simulink model "SCARA_215_ozk"  (R2015a)
settings: Solver=ode1  StartTime=0.0  StopTime=Inf  FixedStep=0.001  RelTol=1e-3
PostLoadFcn:
  | , if any(exist('dsrtsu_mdlpostloadfcn', 'file') == [2, 3, 6]), try dsrtsu_mdlpostloadfcn('Execute', bdroot); catch fprintf('Error in PostLoadFcn (dsrtsu_mdlpostloadfcn) for model "%s":\n %s\n', bdroot, lasterr); end, end,
libraries: rtilib1104 x9, simulink x7, simulink_extras x2
settings Model: DSRTSU_INTERNAL_RTI_VER=460  DSRTSU_INTERNAL_RTI_TYPE=rti1104  DSRTSU_INTERNAL_RTIFPGA=50  Creator=k18p800a  LastModifiedBy=k18p800a
settings OptimizationCC: BlockReduction=off  OptimizeBlockIOStorage=off  BufferReuse=off  GlobalBufferReuse=off  ExpressionFolding=off  LocalBlockOutputs=off
settings HardwareCC: ProdIntDivRoundTo=Zero  ProdEndianess=BigEndian  ProdHWDeviceType=Generic->Custom  TargetIntDivRoundTo=Zero  TargetEndianess=BigEndian  TargetHWDeviceType=Generic->Custom
settings RTWCC: SystemTargetFile=rti1104.tlc  MakeCommand=make_rti  TemplateMakefile=rti1104.tmf  Description=dSPACE DS1104 Hardware Platform
settings STFCustomTargetCC: GenerateSampleERTMain=off  ParMdlRefBuildCompliant=on  GeneratePreprocessorConditionals=Disable all  ERTCustomFileBanners=off  SupportNonInlinedSFcns=on  SupportVariableSizeSignals=off  MATLABClassNameForMDSCustomization=Simulink.SoftwareTarget.GRTCustomization  GRTInterface=on  SystemTargetFile=rti1104.tlc
settings GRTTargetCC: CompOptLevelCompliant=off  ConcurrentExecutionCompliant=off  CombineOutputUpdateFcns=off  MatFileLogging=off  CPPClassGenCompliant=off  GRTInterface=on  ExtModeMexFile=noextcomm

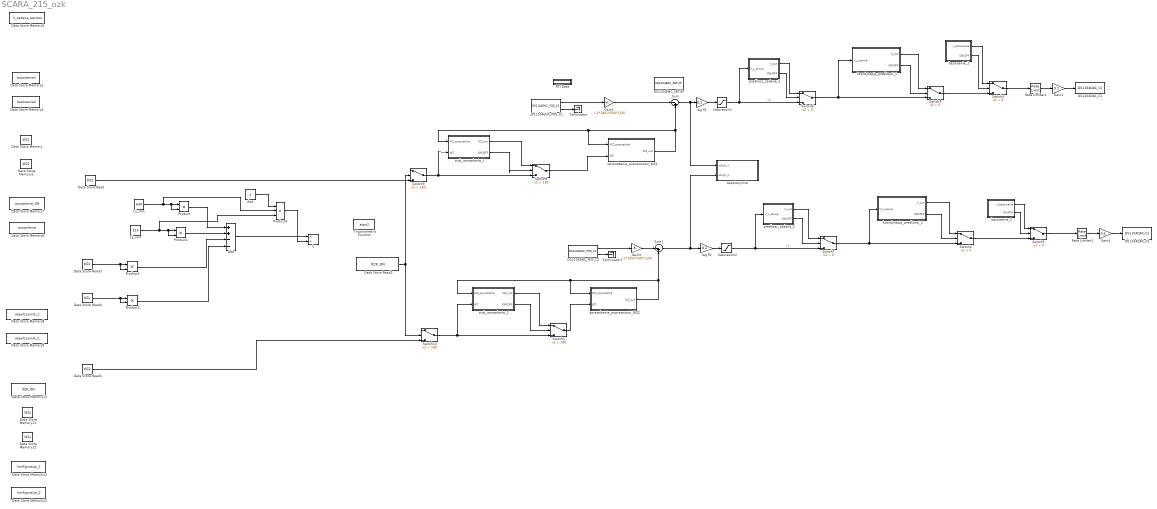
== system SCARA_215_ozk ==
  Add : Sum  Inputs=++--
  DS1104DAC_C1 : rtilib1104/DS1104 MASTER PPC/DS1104DAC_C1  ChannelNo=1  InitValue=0  TermMode=0  TermValue=0  Reserved1=[]  Reserved2=[]  Reserved3=[]  Reserved4=[]  DialogFcn=gui1104dac  UnitName={ 'DS1104DAC_C'}  UnitValues={ 1 }  DSProperties=struct('RTI',struct('Version',uint32(1),'BlockType',struct('isSLSource',uint8(0),'isSLSink',uint8(1),'isHWSource',uint8(0),'isHWSink',uint8(1),'isSetup',uint8(0),'isInline',uint8(1),'isNonInline',uint8(0),'isInterrupt',uint8(0),'isChannelwise',uint8(1)),'IOBoardType','DS1104MASTER','UnitType','DAC','Identifier','DAC','DialogType','ML','BlockSet','NONE','SlaveProcessor','NONE'))
  DS1104DAC_C2 : rtilib1104/DS1104 MASTER PPC/DS1104DAC_C1  ChannelNo=2  InitValue=0  TermMode=0  TermValue=0  Reserved1=[]  Reserved2=[]  Reserved3=[]  Reserved4=[]  DialogFcn=gui1104dac  UnitName={ 'DS1104DAC_C'}  UnitValues={2}  DSProperties=struct('RTI',struct('Version',uint32(1),'BlockType',struct('isSLSource',uint8(0),'isSLSink',uint8(1),'isHWSource',uint8(0),'isHWSink',uint8(1),'isSetup',uint8(0),'isInline',uint8(1),'isNonInline',uint8(0),'isInterrupt',uint8(0),'isChannelwise',uint8(1)),'IOBoardType','DS1104MASTER','UnitType','DAC','Identifier','DAC','DialogType','ML','BlockSet','NONE','SlaveProcessor','NONE'))
  DS1104ENC_POS_C2 : rtilib1104/DS1104 MASTER PPC/DS1104ENC_POS_C1  ChannelNo=2  PosValue=0  Reserved1=[]  Reserved2=[]  Reserved3=[]  Reserved4=[]  DialogFcn=gui1104enc_pos  UnitName={'DS1104ENC_POS_C'}  UnitValues={ 2 }  DSProperties=struct('RTI',struct('Version',uint32(1),'BlockType',struct('isSLSource',uint8(1),'isSLSink',uint8(0),'isHWSource',uint8(1),'isHWSink',uint8(0),'isSetup',uint8(0),'isInline',uint8(1),'isNonInline',uint8(0),'isInterrupt',uint8(0),'isChannelwise',uint8(1)),'IOBoardType','DS1104MASTER','UnitType','ENC','Identifier','ENCPOSCH','DialogType','ML','BlockSet','NONE','SlaveProcessor','NONE'))
  DS1104ENC_SETUP : rtilib1104/DS1104 MASTER PPC/DS1104ENC_SETUP  Reserved1=[]  Reserved2=[]  Reserved3=[]  Reserved4=[]  DialogFcn=gui1104enc_setup  UnitName={'DS1104ENC_SETUP'}  UnitValues={ [] }  DSProperties=struct('RTI',struct('Version',uint32(1),'BlockType',struct('isSLSource',uint8(0),'isSLSink',uint8(0),'isHWSource',uint8(0),'isHWSink',uint8(0),'isSetup',uint8(0),'isInline',uint8(1),'isNonInline',uint8(0),'isInterrupt',uint8(0),'isChannelwise',uint8(0)),'IOBoardType','DS1104MASTER','UnitType','ENC','Identifier','ENCSETUP','DialogType','ML','BlockSet','NONE','SlaveProcessor','NONE'))
      settings: SignalType=[0 0]
  Data Store Memory : DataStoreMemory  DataStoreName=WZ1  ReadBeforeWriteMsg=warning  WriteAfterWriteMsg=warning  WriteAfterReadMsg=warning
  Data Store Memory1 : DataStoreMemory  DataStoreName=WZ2  ReadBeforeWriteMsg=warning  WriteAfterWriteMsg=warning  WriteAfterReadMsg=warning
  Data Store Memory11 : DataStoreMemory  DataStoreName=WZx  ReadBeforeWriteMsg=warning  WriteAfterWriteMsg=warning  WriteAfterReadMsg=warning
  Data Store Memory12 : DataStoreMemory  DataStoreName=WZy  ReadBeforeWriteMsg=warning  WriteAfterWriteMsg=warning  WriteAfterReadMsg=warning
  Data Store Memory13 : DataStoreMemory  DataStoreName=OZK_ON  ReadBeforeWriteMsg=warning  WriteAfterWriteMsg=warning  WriteAfterReadMsg=warning  InitialValue=false  OutDataTypeStr=boolean
  Data Store Memory14 : DataStoreMemory  DataStoreName=konfiguracja_1  ReadBeforeWriteMsg=warning  WriteAfterWriteMsg=warning  WriteAfterReadMsg=warning  InitialValue=false  OutDataTypeStr=boolean
  Data Store Memory15 : DataStoreMemory  DataStoreName=konfiguracja_2  ReadBeforeWriteMsg=warning  WriteAfterWriteMsg=warning  WriteAfterReadMsg=warning  InitialValue=false  OutDataTypeStr=boolean
  Data Store Memory2 : DataStoreMemory  DataStoreName=bazowanie1  ReadBeforeWriteMsg=warning  WriteAfterWriteMsg=warning  WriteAfterReadMsg=warning  InitialValue=false  OutDataTypeStr=boolean
  Data Store Memory3 : DataStoreMemory  DataStoreName=bazowanie2  ReadBeforeWriteMsg=warning  WriteAfterWriteMsg=warning  WriteAfterReadMsg=warning  InitialValue=false  OutDataTypeStr=boolean
  Data Store Memory5 : DataStoreMemory  DataStoreName=V_zadana_wartosc  ReadBeforeWriteMsg=warning  WriteAfterWriteMsg=warning  WriteAfterReadMsg=warning  InitialValue=100  OutDataTypeStr=double
  Data Store Memory6 : DataStoreMemory  DataStoreName=wyzwolenie  ReadBeforeWriteMsg=warning  WriteAfterWriteMsg=warning  WriteAfterReadMsg=warning  InitialValue=false  OutDataTypeStr=boolean
  Data Store Memory7 : DataStoreMemory  DataStoreName=wyzwalanie_ON  ReadBeforeWriteMsg=warning  WriteAfterWriteMsg=warning  WriteAfterReadMsg=warning  InitialValue=false  OutDataTypeStr=boolean
  Data Store Memory8 : DataStoreMemory  DataStoreName=wspolczynnik_1  ReadBeforeWriteMsg=warning  WriteAfterWriteMsg=warning  WriteAfterReadMsg=warning
  Data Store Memory9 : DataStoreMemory  DataStoreName=wspolczynnik_2  ReadBeforeWriteMsg=warning  WriteAfterWriteMsg=warning  WriteAfterReadMsg=warning
  Data Store Read : DataStoreRead  DialogController=Simulink.DDGSource  DataStoreName=WZ1
  Data Store Read1 : DataStoreRead  DataStoreName=WZ2
  Data Store Read2 : DataStoreRead  DataStoreName=OZK_ON
  Data Store Read3 : DataStoreRead  DataStoreName=WZx
  Data Store Read4 : DataStoreRead  DataStoreName=WZy
  Gain1 : Gain  Gain=(-2*180)/(500*128)
  Gain2 : Gain  Gain=0.1
  Gain3 : Gain  Gain=(-2*180)/(500*128)
  Gain4 : Gain  Gain=0.1
  L : Product  Inputs=*/
  L1_mm : Constant  Value=630
  "L2_mm " : Constant  Value=510
  Product{,1..3} (4 alike) : Product
  Product4 : Product  Inputs=3
  RTI Data : Subsystem  Tag=struct('RTIDataServer',struct('RTIDataServerVs','2','RTIModelDescription','struct(''main'',''SCARA_215_ozk'',''sub'',''SCARA_215_ozk'',''isMp'',0)'))  LoadFcn="if exist('rtidc'), try,  rtidc('DataHostBlockClbLoad', gcbh); catch, disp(['Warning: ''LoadFcn'' for RTI Data block failed: ' lasterr]); end, end,"  mask(RTI_DATA_HOST){}
      mask help:
      | RTI Data Block.
      | This block is used by RTI to store internal model-dependent data.
      | Please keep this block on the root level of the model. Deleting this block will result in data loss.
      |
      | NEVER DELETE OR COPY THIS BLOCK!
      settings: CopyFcn="if exist('rtidc'), try,  rtidc('DataHostBlockClbCopy', gcbh); catch, disp(['Warning: ''CopyFcn'' for RTI Data block failed: ' lasterr]); end, end,"  DeleteFcn="if exist('rtidc'), try,  rtidc('DataHostBlockClbDelete', gcbh); catch, disp(['Warning: ''DeleteFcn'' for RTI Data block failed: ' lasterr]); end, end,"  ModelCloseFcn="if exist('rtidc'), try,  rtidc('DataHostBlockClbModelClose', gcbh); catch, disp(['Warning: ''ModelCloseFcn'' for RTI Data block failed: ' lasterr]); end, end,"  PreSaveFcn="if exist('rtidc'), try,  rtidc('DataHostBlockClbPreSave', gcbh); catch, disp(['Warning: ''PreSaveFcn'' for RTI Data block failed: ' lasterr]); end, end,"  PostSaveFcn="if exist('rtidc'), try,  rtidc('DataHostBlockClbPostSave', gcbh); catch, disp(['Warning: ''PostSaveFcn'' for RTI Data block failed: ' lasterr]); end, end,"  NameChangeFcn="if exist('rtidc'), try,  rtidc('DataHostBlockClbNameChange', gcbh); catch, disp(['Warning: ''NameChangeFcn'' for RTI Data block failed: ' lasterr]); end, end,"
      mask Help:
      | RTI Data Block.
      | This block is used by RTI to store internal model-dependent data.
      | Please keep this block on the root level of the model. Deleting this block will result in data loss.
      | 
      | NEVER DELETE OR COPY THIS BLOCK!
      mask Display:
      | text(0.5, 0.5, 'RTI Data', 'HorizontalAlignment', 'center');
      | plot([1 0]);
  Rate Limiter1 : RateLimiter  RisingSlewLimit=50  FallingSlewLimit=-50  SampleTimeMode=inherited
  Rate Limiter2 : RateLimiter  RisingSlewLimit=50  FallingSlewLimit=-50  SampleTimeMode=inherited
  Saturation1 : Saturate  UpperLimit=3  LowerLimit=-3
  Saturation2 : Saturate  UpperLimit=3  LowerLimit=-3
  Sum : Sum  Inputs=|-+
  Sum1 : Sum  Inputs=|-+
  Switch{1,8..10} (4 alike) : Switch  Criteria=u2 > Threshold  Threshold=180
  Switch{2..7} (6 alike) : Switch  Criteria=u2 > Threshold
  Terminator : Terminator
  Terminator1 : Terminator
  Trigonometric Function : Trigonometry  Operator=atan2
  _DS1104ENC_POS_C1 : rtilib1104/DS1104 MASTER PPC/DS1104ENC_POS_C1  ChannelNo=1  PosValue=0  Reserved1=[]  Reserved2=[]  Reserved3=[]  Reserved4=[]  DialogFcn=gui1104enc_pos  UnitName={'DS1104ENC_POS_C'}  UnitValues={ 1 }  DSProperties=struct('RTI',struct('Version',uint32(1),'BlockType',struct('isSLSource',uint8(1),'isSLSink',uint8(0),'isHWSource',uint8(1),'isHWSink',uint8(0),'isSetup',uint8(0),'isInline',uint8(1),'isNonInline',uint8(0),'isInterrupt',uint8(0),'isChannelwise',uint8(1)),'IOBoardType','DS1104MASTER','UnitType','ENC','Identifier','ENCPOSCH','DialogType','ML','BlockSet','NONE','SlaveProcessor','NONE'))
  bazowanie_1 : Subsystem
  "bazowanie_2 " : Subsystem
  dwa : Constant  Value=2
  koordynacja_predkosci_1 : Subsystem
  koordynacja_predkosci_2 : Subsystem
  predkosc_zadana_1 : Subsystem
  predkosc_zadana_2 : Subsystem
  reg P1 : Gain  Gain=0.2
  reg P2 : Gain  Gain=0.2
  sprawdzenie_poprawnosci_WZ1 : Subsystem
  sprawdzenie_poprawnosci_WZ2 : Subsystem
  tryb_wyzwalania_1 : Subsystem
  tryb_wyzwalania_2 : Subsystem
  wspolczynniki : Subsystem
  wires:
  Rate Limiter1/1 -> Gain2/1
  Rate Limiter2/1 -> Gain4/1
  reg P1/1 -> Saturation1/1
  reg P2/1 -> Saturation2/1
  Sum/1 -> wspolczynniki/1(uchyb_1), reg P1/1
  Sum1/1 -> wspolczynniki/2(uchyb_2), reg P2/1
  _DS1104ENC_POS_C1/1 -> Gain1/1
  Gain1/1 -> Sum/1
  DS1104ENC_POS_C2/1 -> Gain3/1
  Gain3/1 -> Sum1/1
  Gain2/1 -> DS1104DAC_C1/1
  Gain4/1 -> DS1104DAC_C2/1
  _DS1104ENC_POS_C1/2 -> Terminator/1
  DS1104ENC_POS_C2/2 -> Terminator1/1
  Switch4/1 -> Rate Limiter1/1
  Switch5/1 -> Rate Limiter2/1
  bazowanie_1/1(v_bazowania) -> Switch4/1
  bazowanie_1/2(ON/OFF) -> Switch4/2
  "bazowanie_2 "/1(v_bazowania) -> Switch5/1
  "bazowanie_2 "/2(On/OFF) -> Switch5/2
  Saturation1/1 -> predkosc_zadana_1/1(V_z_serwa), Switch6/3  "v1"
  predkosc_zadana_1/1(V_out) -> Switch6/1
  predkosc_zadana_1/2(ON/OFF) -> Switch6/2
  Saturation2/1 -> Switch7/3, predkosc_zadana_2/1(V_z_serwa)  "v1"
  predkosc_zadana_2/1(V_out) -> Switch7/1
  predkosc_zadana_2/2(ON/OFF) -> Switch7/2
  tryb_wyzwalania_1/1(WZ_out) -> Switch8/1
  tryb_wyzwalania_1/2(ON/OFF) -> Switch8/2
  sprawdzenie_poprawnosci_WZ1/1(WZ_out) -> Sum/2, tryb_wyzwalania_1/1(WZ_poprzednia), sprawdzenie_poprawnosci_WZ1/1(WZ_poprzednia)
  Switch8/1 -> sprawdzenie_poprawnosci_WZ1/2(WZ)
  tryb_wyzwalania_2/1(WZ_out) -> Switch1/1
  tryb_wyzwalania_2/2(ON/OFF) -> Switch1/2
  sprawdzenie_poprawnosci_WZ2/1(WZ_out) -> Sum1/2, tryb_wyzwalania_2/1(WZ_poprzednia), sprawdzenie_poprawnosci_WZ2/1(WZ_poprzednia)
  Switch1/1 -> sprawdzenie_poprawnosci_WZ2/2(WZ)
  Switch2/1 -> Switch5/3
  Switch7/1 -> koordynacja_predkosci_2/1(V_z_serwa), Switch2/3
  koordynacja_predkosci_2/1(V_out) -> Switch2/1
  koordynacja_predkosci_2/2(ON/OFF) -> Switch2/2
  Switch3/1 -> Switch4/3
  Switch6/1 -> koordynacja_predkosci_1/1(V_z_serwa), Switch3/3
  koordynacja_predkosci_1/1(V_out) -> Switch3/1
  koordynacja_predkosci_1/2(ON/OFF) -> Switch3/2
  Switch9/1 -> tryb_wyzwalania_1/2(WZ), Switch8/3
  Data Store Read/1 -> Switch9/3
  Switch10/1 -> tryb_wyzwalania_2/2(WZ), Switch1/3
  Data Store Read1/1 -> Switch10/3
  Data Store Read2/1 -> Switch9/2, Switch10/2
  L1_mm/1 -> Product4/2, Product/2, Product/1
  "L2_mm "/1 -> Product4/3, Product1/2, Product1/1
  Data Store Read3/1 -> Product2/2, Product2/1
  Data Store Read4/1 -> Product3/2, Product3/1
  Product/1 -> Add/1
  Product1/1 -> Add/2
  Product2/1 -> Add/3
  Product3/1 -> Add/4
  Add/1 -> L/1
  dwa/1 -> Product4/1
  Product4/1 -> L/2

== system SCARA_215_ozk/RTI Data ==
  RTI Data Store : Subsystem  Tag="struct('private',struct('version',struct('dsVer',uint32(2),'dsVerCreation',uint32(2),'RTI',struct('ver','7.4','type','RTI1104')),'access',struct('type','Model','isPerm',1,'created',['26-Mar-2018 08:24:55'],'modified',['16-Apr-2018 08:48:33'],'location','')),'public',struct('main',struct('data',[]),'sub',struct('name',{{'SCARA_215_ozk'}},'data',{{struct('TH',struct('thTaskInfo',struct('taskType',{'TIMER','HWINT','TMRINT','SWINT','GLINT'},'tasksNumOf',{1,0,0,0,0},'srcIds',{{'TIMERA'},{},{},{},{}},'taskNames',{{['Timer Task 1']},{},{},{},{}})),'th_tc',struct('dataType','TASK','taskGroupId','','taskGroupList',{{}},'taskSchedulingPolicy','FCFS','taskType','TIMER','blkh',-1,'srcId','TIMERA','srcSgnName',['Timer A interrupt'],'srcCpuName','','taskName',['Timer Task 1  [0.001] s'],'taskNameDisplayExt','','smplTime',0.001,'smplTimeOffs',0,'hasFixedPriority',0,'priority',1,'hasFixedOvc',0,'ovcType',1,'ovcMax',1),'tc_th',struct('dataType','TASK','taskGroupId','','taskGroupList',{{}},'taskSchedulingPolicy','FCFS','taskType','TIMER','blkh',-1,'srcId','TIMERA','srcSgnName',['Timer A interrupt'],'srcCpuName','','taskName',['Timer Task 1  [0.001] s'],'taskNameDisplayExt','','smplTime',0.001,'smplTimeOffs',0,'hasFixedPriority',0,'priority',1,'hasFixedOvc',0,'ovcType',1,'ovcMax',1))}})))"  mask(RTI_DATA_STORE){}
      mask help:
      | RTI Data Store Block. This block is used by RTI to store internal model dependent data. Deleting this block will result in data loss.
      |
      | NEVER DELETE, COPY, OR MODIFY THIS BLOCK!
      mask Help:
      | RTI Data Store Block. This block is used by RTI to store internal model dependent data. Deleting this block will result in data loss.
      | 
      | NEVER DELETE, COPY, OR MODIFY THIS BLOCK!
      mask Display: text(0.5, 0.5, ' ', 'HorizontalAlignment', 'center');

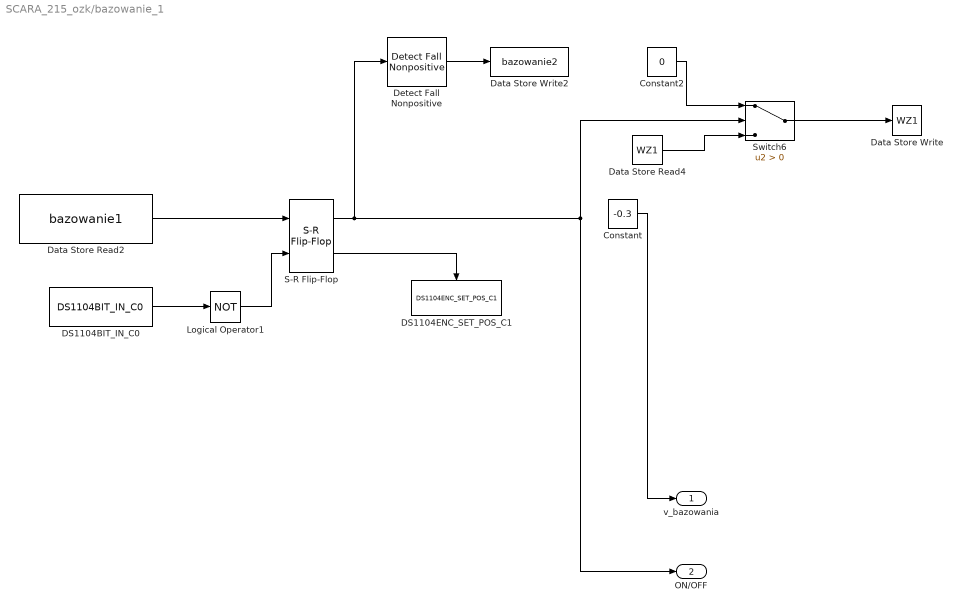
== system SCARA_215_ozk/bazowanie_1 ==
  Constant : Constant  Value=-0.3
  Constant2 : Constant  Value=0
  DS1104BIT_IN_C0 : rtilib1104/DS1104 MASTER PPC/DS1104BIT_IN_C0  ChannelNo=0  Reserved1=[]  Reserved2=[]  Reserved3=[]  Reserved4=[]  DialogFcn=gui1104bit_in  UnitName={'DS1104BIT_IN_C'}  UnitValues={ 0 }  DSProperties=struct('RTI',struct('Version',uint32(1),'BlockType',struct('isSLSource',uint8(1),'isSLSink',uint8(0),'isHWSource',uint8(1),'isHWSink',uint8(0),'isSetup',uint8(0),'isInline',uint8(1),'isNonInline',uint8(0),'isInterrupt',uint8(0),'isChannelwise',uint8(1)),'IOBoardType','DS1104MASTER','UnitType','BIT','Identifier','BITINCH','DialogType','ML','BlockSet','NONE','SlaveProcessor','NONE'))
  DS1104ENC_SET_POS_C1 : rtilib1104/DS1104 MASTER PPC/DS1104ENC_SET_POS_C1  ChannelNo=1  PosValue=0  Reserved1=[]  Reserved2=[]  Reserved3=[]  Reserved4=[]  DialogFcn=gui1104enc_set_pos  UnitName={'DS1104ENC_SET_POS_C'}  UnitValues={ 1 }  DSProperties=struct('RTI',struct('Version',uint32(1),'BlockType',struct('isSLSource',uint8(0),'isSLSink',uint8(1),'isHWSource',uint8(0),'isHWSink',uint8(1),'isSetup',uint8(0),'isInline',uint8(1),'isNonInline',uint8(0),'isInterrupt',uint8(0),'isChannelwise',uint8(1)),'IOBoardType','DS1104MASTER','UnitType','ENC','Identifier','ENCRESET','DialogType','ML','BlockSet','NONE','SlaveProcessor','NONE'))
  Data Store Read2 : DataStoreRead  DataStoreName=bazowanie1
  Data Store Read4 : DataStoreRead  DialogController=Simulink.DDGSource  DataStoreName=WZ1
  Data Store Write : DataStoreWrite  DataStoreName=WZ1
  Data Store Write2 : DataStoreWrite  DataStoreName=bazowanie2
  Detect Fall Nonpositive : simulink/Logic and Bit Operations/Detect Fall Nonpositive  vinit=1  InputProcessing=Inherited  OutDataTypeStr=boolean
  Logical Operator1 : Logic  Operator=NOT  AllPortsSameDT=off  OutDataTypeStr=boolean
  S-R Flip-Flop : simulink_extras/Flip Flops/S-R Flip-Flop  initial_condition=0
  Switch6 : Switch  Criteria=u2 > Threshold
  v_bazowania : Outport
  ON/OFF : Outport  Port=2
  wires:
  Constant/1 -> v_bazowania/1
  S-R Flip-Flop/2 -> DS1104ENC_SET_POS_C1/Trigger
  Data Store Read2/1 -> S-R Flip-Flop/1
  S-R Flip-Flop/1 -> ON/OFF/1, Switch6/2, Detect Fall Nonpositive/1
  Logical Operator1/1 -> S-R Flip-Flop/2
  DS1104BIT_IN_C0/1 -> Logical Operator1/1
  Data Store Read4/1 -> Switch6/3
  Constant2/1 -> Switch6/1
  Switch6/1 -> Data Store Write/1
  Detect Fall Nonpositive/1 -> Data Store Write2/1

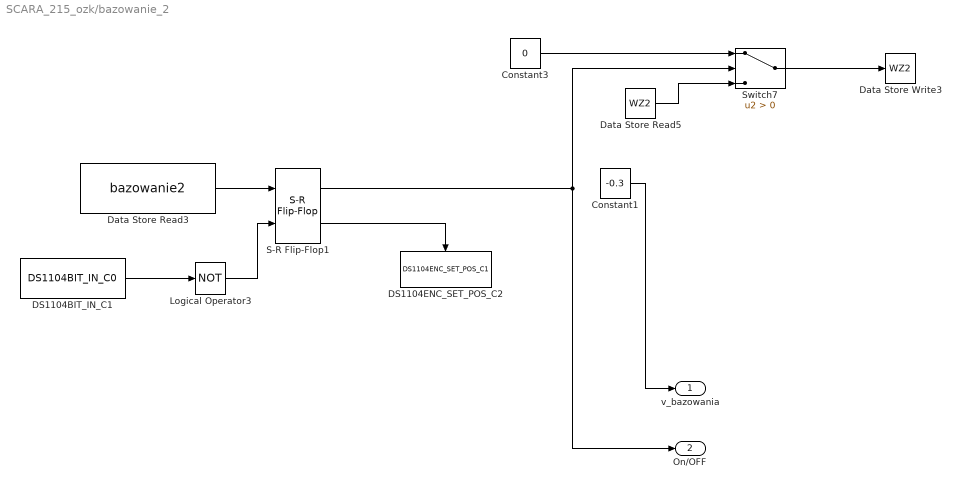
== system SCARA_215_ozk/bazowanie_2  ==
  Constant1 : Constant  Value=-0.3
  Constant3 : Constant  Value=0
  DS1104BIT_IN_C1 : rtilib1104/DS1104 MASTER PPC/DS1104BIT_IN_C0  ChannelNo=1  Reserved1=[]  Reserved2=[]  Reserved3=[]  Reserved4=[]  DialogFcn=gui1104bit_in  UnitName={'DS1104BIT_IN_C'}  UnitValues={ 1 }  DSProperties=struct('RTI',struct('Version',uint32(1),'BlockType',struct('isSLSource',uint8(1),'isSLSink',uint8(0),'isHWSource',uint8(1),'isHWSink',uint8(0),'isSetup',uint8(0),'isInline',uint8(1),'isNonInline',uint8(0),'isInterrupt',uint8(0),'isChannelwise',uint8(1)),'IOBoardType','DS1104MASTER','UnitType','BIT','Identifier','BITINCH','DialogType','ML','BlockSet','NONE','SlaveProcessor','NONE'))
  DS1104ENC_SET_POS_C2 : rtilib1104/DS1104 MASTER PPC/DS1104ENC_SET_POS_C1  ChannelNo=2  PosValue=0  Reserved1=[]  Reserved2=[]  Reserved3=[]  Reserved4=[]  DialogFcn=gui1104enc_set_pos  UnitName={'DS1104ENC_SET_POS_C'}  UnitValues={2}  DSProperties=struct('RTI',struct('Version',uint32(1),'BlockType',struct('isSLSource',uint8(0),'isSLSink',uint8(1),'isHWSource',uint8(0),'isHWSink',uint8(1),'isSetup',uint8(0),'isInline',uint8(1),'isNonInline',uint8(0),'isInterrupt',uint8(0),'isChannelwise',uint8(1)),'IOBoardType','DS1104MASTER','UnitType','ENC','Identifier','ENCRESET','DialogType','ML','BlockSet','NONE','SlaveProcessor','NONE'))
  Data Store Read3 : DataStoreRead  DataStoreName=bazowanie2
  Data Store Read5 : DataStoreRead  DialogController=Simulink.DDGSource  DataStoreName=WZ2
  Data Store Write3 : DataStoreWrite  DataStoreName=WZ2
  Logical Operator3 : Logic  Operator=NOT  AllPortsSameDT=off  OutDataTypeStr=boolean
  S-R Flip-Flop1 : simulink_extras/Flip Flops/S-R Flip-Flop  initial_condition=0
  Switch7 : Switch  Criteria=u2 > Threshold
  v_bazowania : Outport
  On/OFF : Outport  Port=2
  wires:
  Constant1/1 -> v_bazowania/1
  S-R Flip-Flop1/2 -> DS1104ENC_SET_POS_C2/Trigger
  Data Store Read3/1 -> S-R Flip-Flop1/1
  Logical Operator3/1 -> S-R Flip-Flop1/2
  DS1104BIT_IN_C1/1 -> Logical Operator3/1
  Data Store Read5/1 -> Switch7/3
  Constant3/1 -> Switch7/1
  Switch7/1 -> Data Store Write3/1
  S-R Flip-Flop1/1 -> On/OFF/1, Switch7/2

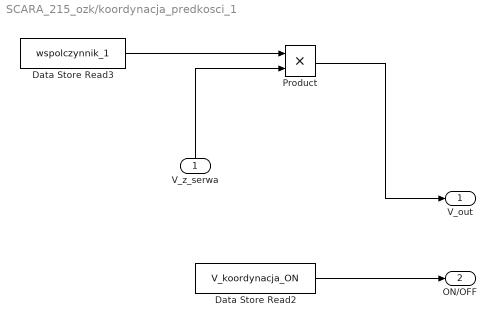
== system SCARA_215_ozk/koordynacja_predkosci_1 ==
  V_z_serwa : Inport
  Data Store Read2 : DataStoreRead  DataStoreName=V_koordynacja_ON
  Data Store Read3 : DataStoreRead  DataStoreName=wspolczynnik_1
  Product : Product
  V_out : Outport
  ON/OFF : Outport  Port=2
  wires:
  Product/1 -> V_out/1
  V_z_serwa/1 -> Product/2
  Data Store Read3/1 -> Product/1
  Data Store Read2/1 -> ON/OFF/1

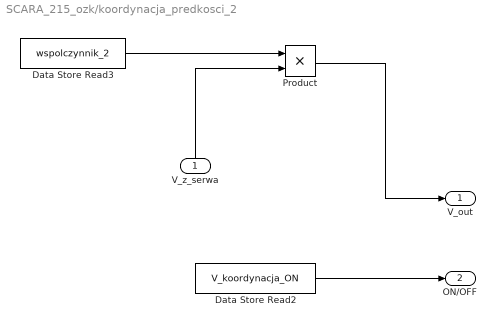
== system SCARA_215_ozk/koordynacja_predkosci_2 ==
  V_z_serwa : Inport
  Data Store Read2 : DataStoreRead  DataStoreName=V_koordynacja_ON
  Data Store Read3 : DataStoreRead  DataStoreName=wspolczynnik_2
  Product : Product
  V_out : Outport
  ON/OFF : Outport  Port=2
  wires:
  Product/1 -> V_out/1
  V_z_serwa/1 -> Product/2
  Data Store Read3/1 -> Product/1
  Data Store Read2/1 -> ON/OFF/1

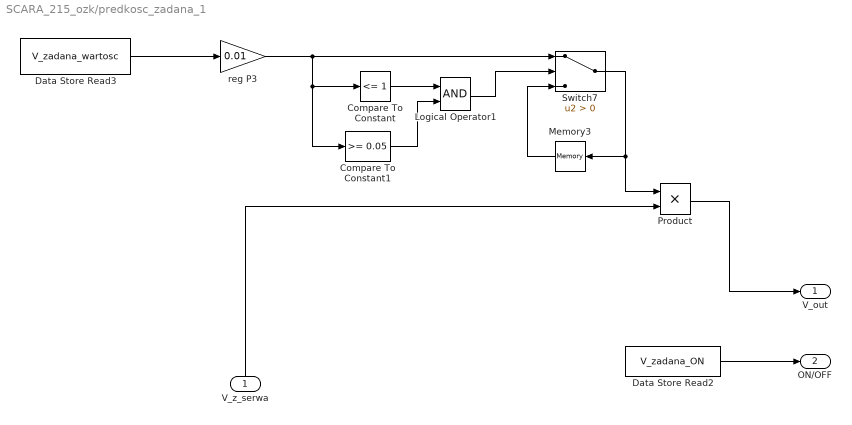
== system SCARA_215_ozk/predkosc_zadana_1 ==
  V_z_serwa : Inport
  Compare To Constant : simulink/Logic and Bit Operations/Compare To Constant  relop=<=  const=1  OutDataTypeStr=boolean
  Compare To Constant1 : simulink/Logic and Bit Operations/Compare To Constant  relop=>=  const=0.05  OutDataTypeStr=boolean
  Data Store Read2 : DataStoreRead  DialogController=Simulink.DDGSource  DataStoreName=V_zadana_ON
  Data Store Read3 : DataStoreRead  DialogController=Simulink.DDGSource  DataStoreName=V_zadana_wartosc
  Logical Operator1 : Logic  AllPortsSameDT=off  OutDataTypeStr=boolean
  Memory3 : Memory  X0=1
  Product : Product
  Switch7 : Switch  Criteria=u2 > Threshold
  reg P3 : Gain  Gain=0.01
  V_out : Outport
  ON/OFF : Outport  Port=2
  wires:
  Logical Operator1/1 -> Switch7/2
  V_z_serwa/1 -> Product/2
  Product/1 -> V_out/1
  Switch7/1 -> Product/1, Memory3/1
  Memory3/1 -> Switch7/3
  reg P3/1 -> Compare To Constant1/1, Compare To Constant/1, Switch7/1
  Compare To Constant1/1 -> Logical Operator1/2
  Compare To Constant/1 -> Logical Operator1/1
  Data Store Read2/1 -> ON/OFF/1
  Data Store Read3/1 -> reg P3/1

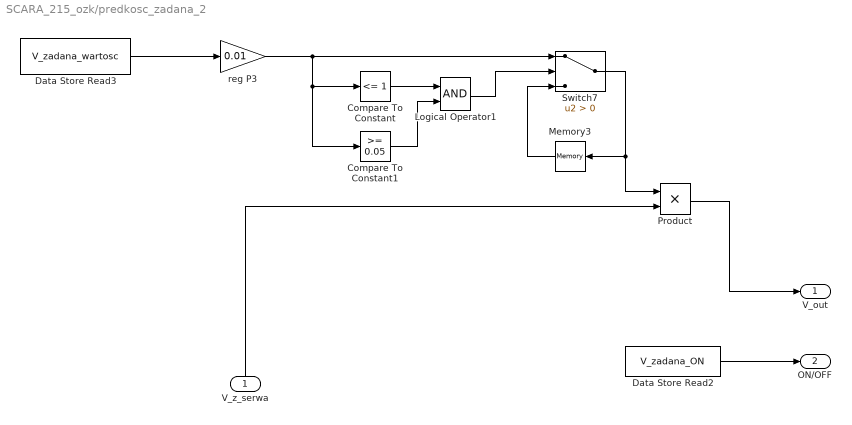
== system SCARA_215_ozk/predkosc_zadana_2 ==
  V_z_serwa : Inport
  Compare To Constant : simulink/Logic and Bit Operations/Compare To Constant  relop=<=  const=1  OutDataTypeStr=boolean
  Compare To Constant1 : simulink/Logic and Bit Operations/Compare To Constant  relop=>=  const=0.05  OutDataTypeStr=boolean
  Data Store Read2 : DataStoreRead  DialogController=Simulink.DDGSource  DataStoreName=V_zadana_ON
  Data Store Read3 : DataStoreRead  DialogController=Simulink.DDGSource  DataStoreName=V_zadana_wartosc
  Logical Operator1 : Logic  AllPortsSameDT=off  OutDataTypeStr=boolean
  Memory3 : Memory  X0=1
  Product : Product
  Switch7 : Switch  Criteria=u2 > Threshold
  reg P3 : Gain  Gain=0.01
  V_out : Outport
  ON/OFF : Outport  Port=2
  wires:
  Logical Operator1/1 -> Switch7/2
  V_z_serwa/1 -> Product/2
  Product/1 -> V_out/1
  Switch7/1 -> Product/1, Memory3/1
  Memory3/1 -> Switch7/3
  reg P3/1 -> Compare To Constant1/1, Compare To Constant/1, Switch7/1
  Compare To Constant1/1 -> Logical Operator1/2
  Compare To Constant/1 -> Logical Operator1/1
  Data Store Read2/1 -> ON/OFF/1
  Data Store Read3/1 -> reg P3/1

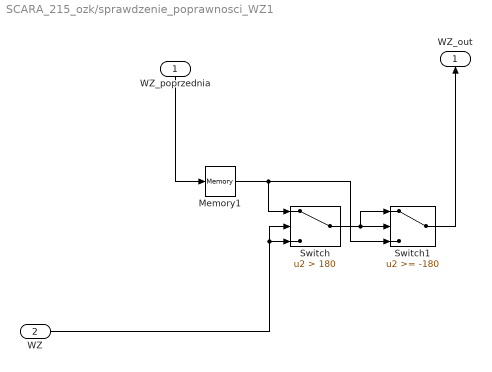
== system SCARA_215_ozk/sprawdzenie_poprawnosci_WZ1 ==
  WZ_poprzednia : Inport
  WZ : Inport  Port=2
  Memory1 : Memory
  Switch : Switch  Criteria=u2 > Threshold  Threshold=180
  Switch1 : Switch  Threshold=-180
  WZ_out : Outport
  wires:
  WZ/1 -> Switch/2, Switch/3
  WZ_poprzednia/1 -> Memory1/1
  Switch/1 -> Switch1/1, Switch1/2
  Switch1/1 -> WZ_out/1
  Memory1/1 -> Switch1/3, Switch/1

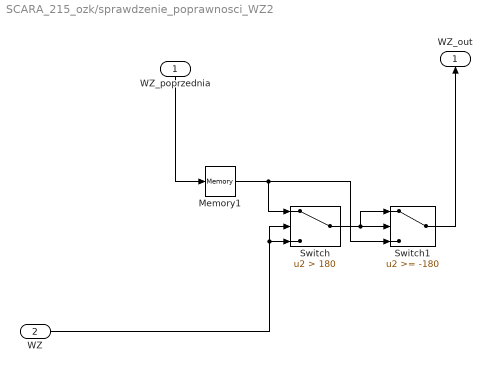
== system SCARA_215_ozk/sprawdzenie_poprawnosci_WZ2 ==
  WZ_poprzednia : Inport
  WZ : Inport  Port=2
  Memory1 : Memory
  Switch : Switch  Criteria=u2 > Threshold  Threshold=180
  Switch1 : Switch  Threshold=-180
  WZ_out : Outport
  wires:
  WZ/1 -> Switch/2, Switch/3
  WZ_poprzednia/1 -> Memory1/1
  Switch/1 -> Switch1/1, Switch1/2
  Switch1/1 -> WZ_out/1
  Memory1/1 -> Switch1/3, Switch/1

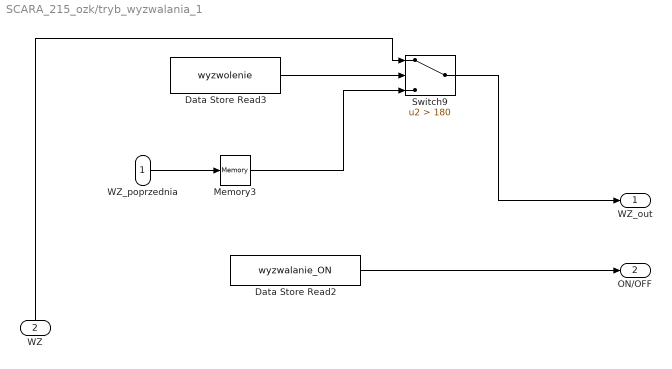
== system SCARA_215_ozk/tryb_wyzwalania_1 ==
  WZ_poprzednia : Inport
  WZ : Inport  Port=2
  Data Store Read2 : DataStoreRead  DataStoreName=wyzwalanie_ON
  Data Store Read3 : DataStoreRead  DataStoreName=wyzwolenie
  Memory3 : Memory
  Switch9 : Switch  Criteria=u2 > Threshold  Threshold=180
  WZ_out : Outport
  ON/OFF : Outport  Port=2
  wires:
  Data Store Read3/1 -> Switch9/2
  Data Store Read2/1 -> ON/OFF/1
  Switch9/1 -> WZ_out/1
  WZ_poprzednia/1 -> Memory3/1
  Memory3/1 -> Switch9/3
  WZ/1 -> Switch9/1

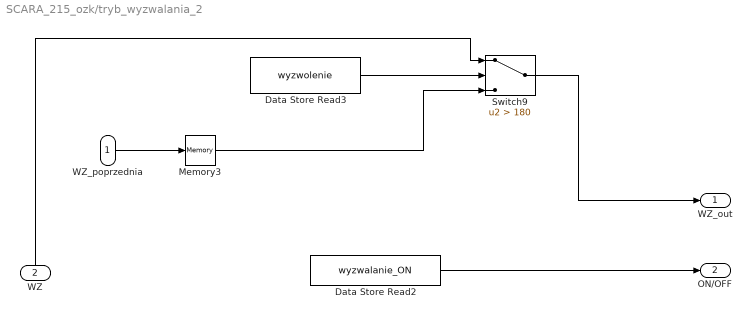
== system SCARA_215_ozk/tryb_wyzwalania_2 ==
  WZ_poprzednia : Inport
  WZ : Inport  Port=2
  Data Store Read2 : DataStoreRead  DataStoreName=wyzwalanie_ON
  Data Store Read3 : DataStoreRead  DataStoreName=wyzwolenie
  Memory3 : Memory
  Switch9 : Switch  Criteria=u2 > Threshold  Threshold=180
  WZ_out : Outport
  ON/OFF : Outport  Port=2
  wires:
  Data Store Read3/1 -> Switch9/2
  Data Store Read2/1 -> ON/OFF/1
  Switch9/1 -> WZ_out/1
  WZ_poprzednia/1 -> Memory3/1
  Memory3/1 -> Switch9/3
  WZ/1 -> Switch9/1

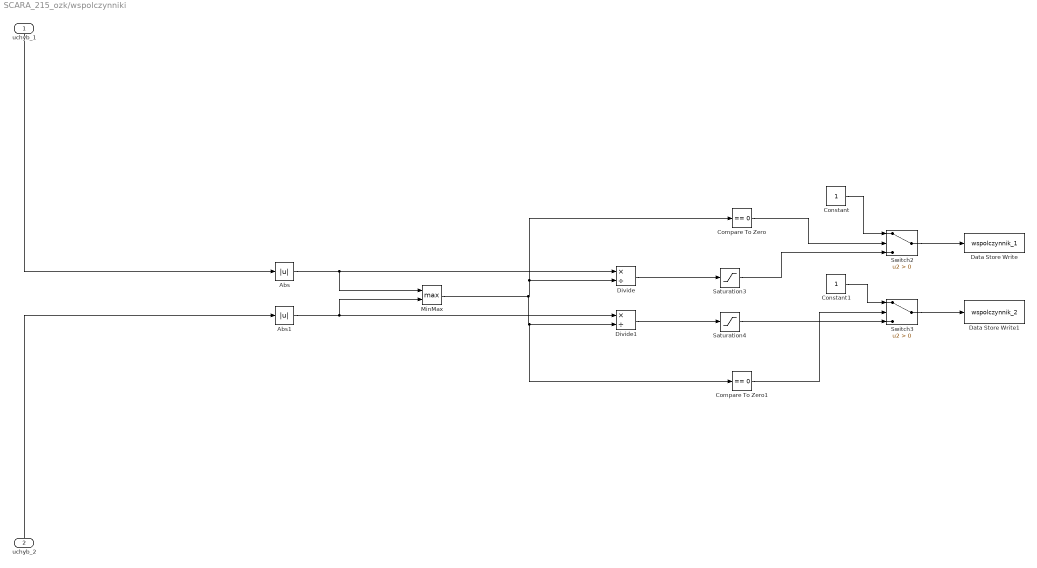
== system SCARA_215_ozk/wspolczynniki ==
  uchyb_1 : Inport
  uchyb_2 : Inport  Port=2
  Abs : Abs
  Abs1 : Abs
  Compare To Zero : simulink/Logic and Bit Operations/Compare To Zero  relop===  OutDataTypeStr=boolean
  Compare To Zero1 : simulink/Logic and Bit Operations/Compare To Zero  relop===  OutDataTypeStr=boolean
  Constant : Constant
  Constant1 : Constant
  Data Store Write : DataStoreWrite  DataStoreName=wspolczynnik_1
  Data Store Write1 : DataStoreWrite  DataStoreName=wspolczynnik_2
  Divide : Product  Inputs=*/
  Divide1 : Product  Inputs=*/
  MinMax : MinMax  Function=max  Inputs=2
  Saturation3 : Saturate  UpperLimit=1  LowerLimit=0.05
  Saturation4 : Saturate  UpperLimit=1  LowerLimit=0.05
  Switch2 : Switch  Criteria=u2 > Threshold
  Switch3 : Switch  Criteria=u2 > Threshold
  wires:
  Compare To Zero/1 -> Switch2/2
  Compare To Zero1/1 -> Switch3/2
  Abs1/1 -> Divide1/1, MinMax/2
  Switch2/1 -> Data Store Write/1
  uchyb_2/1 -> Abs1/1
  uchyb_1/1 -> Abs/1
  MinMax/1 -> Compare To Zero1/1, Divide1/2, Compare To Zero/1, Divide/2
  Switch3/1 -> Data Store Write1/1
  Abs/1 -> Divide/1, MinMax/1
  Constant1/1 -> Switch3/1
  Saturation3/1 -> Switch2/3
  Constant/1 -> Switch2/1
  Saturation4/1 -> Switch3/3
  Divide/1 -> Saturation3/1
  Divide1/1 -> Saturation4/1

== system SCARA_215_ozk/RTI Data/RTI Data Store ==
  RTI Data Store : Subsystem  mask(RTI_DATA_STORE){}
      mask help:
      | RTI Data Store Block. This block is used by RTI to store internal model dependent data. Deleting this block will result in data loss.
      |
      | NEVER DELETE, COPY, OR MODIFY THIS BLOCK!
      mask Help:
      | RTI Data Store Block. This block is used by RTI to store internal model dependent data. Deleting this block will result in data loss.
      | 
      | NEVER DELETE, COPY, OR MODIFY THIS BLOCK!
      mask Display: text(0.5, 0.5, ' ', 'HorizontalAlignment', 'center');

== system SCARA_215_ozk/RTI Data/RTI Data Store/RTI Data Store ==
  RTI Data Store : Subsystem  mask(RTI_DATA_STORE){}
      mask help:
      | RTI Data Store Block. This block is used by RTI to store internal model dependent data. Deleting this block will result in data loss.
      |
      | NEVER DELETE, COPY, OR MODIFY THIS BLOCK!
      mask Help:
      | RTI Data Store Block. This block is used by RTI to store internal model dependent data. Deleting this block will result in data loss.
      | 
      | NEVER DELETE, COPY, OR MODIFY THIS BLOCK!
      mask Display: text(0.5, 0.5, ' ', 'HorizontalAlignment', 'center');

== system SCARA_215_ozk/RTI Data/RTI Data Store/RTI Data Store/RTI Data Store ==
  RTI Data Store : Subsystem  mask(RTI_DATA_STORE){}
      mask help:
      | RTI Data Store Block. This block is used by RTI to store internal model dependent data. Deleting this block will result in data loss.
      |
      | NEVER DELETE, COPY, OR MODIFY THIS BLOCK!
      mask Help:
      | RTI Data Store Block. This block is used by RTI to store internal model dependent data. Deleting this block will result in data loss.
      | 
      | NEVER DELETE, COPY, OR MODIFY THIS BLOCK!
      mask Display: text(0.5, 0.5, ' ', 'HorizontalAlignment', 'center');

== system SCARA_215_ozk/RTI Data/RTI Data Store/RTI Data Store/RTI Data Store/RTI Data Store ==
